simulink library "Nibble_Multiplexers_Lib"  (Simulink 8.7)
settings: Solver=ode45  StartTime=0.0  StopTime=10.0  RelTol=1e-3
libraries: Bit_Multiplexers_Lib x20, commutil2 x16
(part 2 of 2)

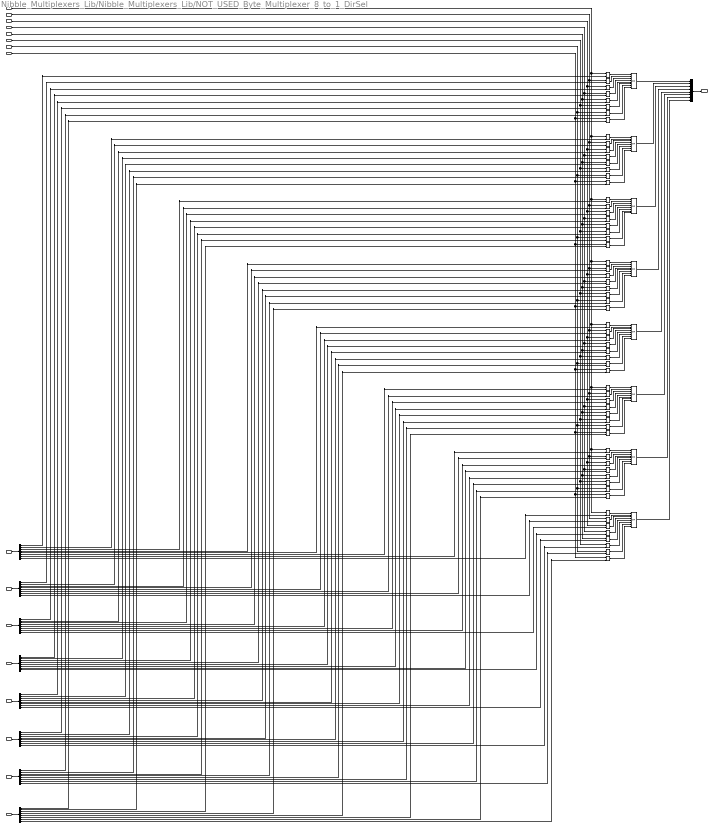
== system Nibble_Multiplexers_Lib/Nibble_Multiplexers_Lib/NOT_USED_Byte_Multiplexer_8_to_1_DirSel ==
  note: Bit_Multiplexer_8_to_1_DirSel(Bit_7)
  note: Bit_Multiplexer_8_to_1_DirSel(Bit_6)
  note: Bit_Multiplexer_8_to_1_DirSel(Bit_5)
  note: Bit_Multiplexer_8_to_1_DirSel(Bit_4)
  note: Bit_Multiplexer_8_to_1_DirSel(Bit_3)
  note: Bit_Multiplexer_8_to_1_DirSel(Bit_2)
  note: Bit_Multiplexer_8_to_1_DirSel(Bit_1)
  note: Bit_Multiplexer_8_to_1_DirSel(Bit_0)
  Select_7(1b) : Inport
  Select_6(1b) : Inport  Port=2
  Select_5(1b) : Inport  Port=3
  Select_4(1b) : Inport  Port=4
  Select_3(1b) : Inport  Port=5
  Select_2(1b) : Inport  Port=6
  Select_1(1b) : Inport  Port=7
  Select_0(1b) : Inport  Port=8
  Data_7(1B) : Inport  Port=9
  Data_6(1B) : Inport  Port=10
  Data_5(1B) : Inport  Port=11
  Data_4(1B) : Inport  Port=12
  Data_3(1B) : Inport  Port=13
  Data_2(1B) : Inport  Port=14
  Data_1(1B) : Inport  Port=15
  Data_0(1B) : Inport  Port=16
  Bus Creator : BusCreator  Inputs=8
  Bus Selector{1..8} (8 alike) : BusSelector  OutputSignals=signal1,signal2,signal3,signal4,signal5,signal6,signal7,signal8
  Logical Operator{,1..7,9..16,18..24,26..33,35..42,44..51,53..60,62..69,71} (64 alike) : Logic  IconShape=distinctive  AllPortsSameDT=off  OutDataTypeStr=boolean
  Logical Operator{8,17,25,34,43,52,61,70} (8 alike) : Logic  Operator=OR  Inputs=8  IconShape=distinctive  OutDataTypeStr=boolean
  Data(1B) : Outport
  wires:
  Data_7(1B)/1 -> Bus Selector7/1
  Bus Creator/1 -> Data(1B)/1
  Bus Selector8/8 -> Logical Operator69/2  "<signal8>"
  Bus Selector6/8 -> Logical Operator68/2  "<signal8>"
  Bus Selector5/8 -> Logical Operator67/2  "<signal8>"
  Bus Selector4/8 -> Logical Operator66/2  "<signal8>"
  Bus Selector3/8 -> Logical Operator65/2  "<signal8>"
  Bus Selector2/8 -> Logical Operator64/2  "<signal8>"
  Bus Selector1/8 -> Logical Operator63/2  "<signal8>"
  Bus Selector7/8 -> Logical Operator71/2  "<signal8>"
  Bus Selector8/7 -> Logical Operator60/2  "<signal7>"
  Bus Selector6/7 -> Logical Operator59/2  "<signal7>"
  Bus Selector5/7 -> Logical Operator58/2  "<signal7>"
  Bus Selector4/7 -> Logical Operator57/2  "<signal7>"
  Bus Selector3/7 -> Logical Operator56/2  "<signal7>"
  Bus Selector2/7 -> Logical Operator55/2  "<signal7>"
  Bus Selector1/7 -> Logical Operator54/2  "<signal7>"
  Bus Selector7/7 -> Logical Operator62/2  "<signal7>"
  Bus Selector8/6 -> Logical Operator51/2  "<signal6>"
  Bus Selector6/6 -> Logical Operator50/2  "<signal6>"
  Bus Selector5/6 -> Logical Operator49/2  "<signal6>"
  Bus Selector4/6 -> Logical Operator48/2  "<signal6>"
  Bus Selector3/6 -> Logical Operator47/2  "<signal6>"
  Bus Selector2/6 -> Logical Operator46/2  "<signal6>"
  Bus Selector1/6 -> Logical Operator45/2  "<signal6>"
  Bus Selector7/6 -> Logical Operator53/2  "<signal6>"
  Bus Selector8/5 -> Logical Operator42/2  "<signal5>"
  Bus Selector6/5 -> Logical Operator41/2  "<signal5>"
  Bus Selector5/5 -> Logical Operator40/2  "<signal5>"
  Bus Selector4/5 -> Logical Operator39/2  "<signal5>"
  Bus Selector3/5 -> Logical Operator38/2  "<signal5>"
  Bus Selector2/5 -> Logical Operator37/2  "<signal5>"
  Bus Selector1/5 -> Logical Operator36/2  "<signal5>"
  Bus Selector7/5 -> Logical Operator44/2  "<signal5>"
  Bus Selector8/4 -> Logical Operator33/2  "<signal4>"
  Bus Selector6/4 -> Logical Operator32/2  "<signal4>"
  Bus Selector5/4 -> Logical Operator31/2  "<signal4>"
  Bus Selector4/4 -> Logical Operator30/2  "<signal4>"
  Bus Selector3/4 -> Logical Operator29/2  "<signal4>"
  Bus Selector2/4 -> Logical Operator28/2  "<signal4>"
  Bus Selector1/4 -> Logical Operator27/2  "<signal4>"
  Bus Selector7/4 -> Logical Operator35/2  "<signal4>"
  Bus Selector8/3 -> Logical Operator24/2  "<signal3>"
  Bus Selector6/3 -> Logical Operator23/2  "<signal3>"
  Bus Selector5/3 -> Logical Operator22/2  "<signal3>"
  Bus Selector4/3 -> Logical Operator21/2  "<signal3>"
  Bus Selector3/3 -> Logical Operator20/2  "<signal3>"
  Bus Selector2/3 -> Logical Operator19/2  "<signal3>"
  Bus Selector1/3 -> Logical Operator18/2  "<signal3>"
  Bus Selector7/3 -> Logical Operator26/2  "<signal3>"
  Bus Selector8/2 -> Logical Operator16/2  "<signal2>"
  Bus Selector6/2 -> Logical Operator15/2  "<signal2>"
  Bus Selector5/2 -> Logical Operator14/2  "<signal2>"
  Bus Selector4/2 -> Logical Operator13/2  "<signal2>"
  Bus Selector3/2 -> Logical Operator12/2  "<signal2>"
  Bus Selector2/2 -> Logical Operator11/2  "<signal2>"
  Bus Selector1/2 -> Logical Operator10/2  "<signal2>"
  Bus Selector7/2 -> Logical Operator9/2  "<signal2>"
  Bus Selector8/1 -> Logical Operator7/2  "<signal1>"
  Bus Selector6/1 -> Logical Operator6/2  "<signal1>"
  Bus Selector5/1 -> Logical Operator5/2  "<signal1>"
  Bus Selector4/1 -> Logical Operator4/2  "<signal1>"
  Bus Selector3/1 -> Logical Operator3/2  "<signal1>"
  Bus Selector2/1 -> Logical Operator2/2  "<signal1>"
  Bus Selector1/1 -> Logical Operator1/2  "<signal1>"
  Bus Selector7/1 -> Logical Operator/2  "<signal1>"
  Select_7(1b)/1 -> Logical Operator44/1, Logical Operator53/1, Logical Operator62/1, Logical Operator71/1, Logical Operator35/1, Logical Operator26/1, Logical Operator9/1, Logical Operator/1
  Select_6(1b)/1 -> Logical Operator36/1, Logical Operator45/1, Logical Operator54/1, Logical Operator63/1, Logical Operator27/1, Logical Operator18/1, Logical Operator10/1, Logical Operator1/1
  Select_4(1b)/1 -> Logical Operator38/1, Logical Operator47/1, Logical Operator56/1, Logical Operator65/1, Logical Operator29/1, Logical Operator20/1, Logical Operator12/1, Logical Operator3/1
  Select_3(1b)/1 -> Logical Operator39/1, Logical Operator48/1, Logical Operator57/1, Logical Operator66/1, Logical Operator30/1, Logical Operator21/1, Logical Operator13/1, Logical Operator4/1
  Select_2(1b)/1 -> Logical Operator40/1, Logical Operator49/1, Logical Operator58/1, Logical Operator67/1, Logical Operator31/1, Logical Operator22/1, Logical Operator14/1, Logical Operator5/1
  Select_0(1b)/1 -> Logical Operator42/1, Logical Operator51/1, Logical Operator60/1, Logical Operator69/1, Logical Operator33/1, Logical Operator24/1, Logical Operator16/1, Logical Operator7/1
  Logical Operator17/1 -> Bus Creator/2
  Logical Operator34/1 -> Bus Creator/4
  Logical Operator52/1 -> Bus Creator/6
  Logical Operator70/1 -> Bus Creator/8
  Select_1(1b)/1 -> Logical Operator41/1, Logical Operator50/1, Logical Operator59/1, Logical Operator68/1, Logical Operator32/1, Logical Operator23/1, Logical Operator15/1, Logical Operator6/1
  Select_5(1b)/1 -> Logical Operator37/1, Logical Operator46/1, Logical Operator55/1, Logical Operator64/1, Logical Operator28/1, Logical Operator19/1, Logical Operator11/1, Logical Operator2/1
  Logical Operator61/1 -> Bus Creator/7
  Logical Operator43/1 -> Bus Creator/5
  Logical Operator25/1 -> Bus Creator/3
  Logical Operator8/1 -> Bus Creator/1
  Logical Operator3/1 -> Logical Operator8/4
  Logical Operator2/1 -> Logical Operator8/3
  Logical Operator1/1 -> Logical Operator8/2
  Logical Operator/1 -> Logical Operator8/1
  Logical Operator7/1 -> Logical Operator8/8
  Logical Operator6/1 -> Logical Operator8/7
  Logical Operator5/1 -> Logical Operator8/6
  Logical Operator4/1 -> Logical Operator8/5
  Logical Operator12/1 -> Logical Operator17/4
  Logical Operator11/1 -> Logical Operator17/3
  Logical Operator10/1 -> Logical Operator17/2
  Logical Operator9/1 -> Logical Operator17/1
  Logical Operator16/1 -> Logical Operator17/8
  Logical Operator15/1 -> Logical Operator17/7
  Logical Operator14/1 -> Logical Operator17/6
  Logical Operator13/1 -> Logical Operator17/5
  Logical Operator20/1 -> Logical Operator25/4
  Logical Operator19/1 -> Logical Operator25/3
  Logical Operator18/1 -> Logical Operator25/2
  Logical Operator26/1 -> Logical Operator25/1
  Logical Operator24/1 -> Logical Operator25/8
  Logical Operator23/1 -> Logical Operator25/7
  Logical Operator22/1 -> Logical Operator25/6
  Logical Operator21/1 -> Logical Operator25/5
  Logical Operator29/1 -> Logical Operator34/4
  Logical Operator28/1 -> Logical Operator34/3
  Logical Operator27/1 -> Logical Operator34/2
  Logical Operator35/1 -> Logical Operator34/1
  Logical Operator33/1 -> Logical Operator34/8
  Logical Operator32/1 -> Logical Operator34/7
  Logical Operator31/1 -> Logical Operator34/6
  Logical Operator30/1 -> Logical Operator34/5
  Logical Operator38/1 -> Logical Operator43/4
  Logical Operator37/1 -> Logical Operator43/3
  Logical Operator36/1 -> Logical Operator43/2
  Logical Operator44/1 -> Logical Operator43/1
  Logical Operator42/1 -> Logical Operator43/8
  Logical Operator41/1 -> Logical Operator43/7
  Logical Operator40/1 -> Logical Operator43/6
  Logical Operator39/1 -> Logical Operator43/5
  Logical Operator47/1 -> Logical Operator52/4
  Logical Operator46/1 -> Logical Operator52/3
  Logical Operator45/1 -> Logical Operator52/2
  Logical Operator53/1 -> Logical Operator52/1
  Logical Operator51/1 -> Logical Operator52/8
  Logical Operator50/1 -> Logical Operator52/7
  Logical Operator49/1 -> Logical Operator52/6
  Logical Operator48/1 -> Logical Operator52/5
  Logical Operator56/1 -> Logical Operator61/4
  Logical Operator55/1 -> Logical Operator61/3
  Logical Operator54/1 -> Logical Operator61/2
  Logical Operator62/1 -> Logical Operator61/1
  Logical Operator60/1 -> Logical Operator61/8
  Logical Operator59/1 -> Logical Operator61/7
  Logical Operator58/1 -> Logical Operator61/6
  Logical Operator57/1 -> Logical Operator61/5
  Logical Operator65/1 -> Logical Operator70/4
  Logical Operator64/1 -> Logical Operator70/3
  Logical Operator63/1 -> Logical Operator70/2
  Logical Operator71/1 -> Logical Operator70/1
  Logical Operator69/1 -> Logical Operator70/8
  Logical Operator68/1 -> Logical Operator70/7
  Logical Operator67/1 -> Logical Operator70/6
  Logical Operator66/1 -> Logical Operator70/5
  Data_0(1B)/1 -> Bus Selector8/1
  Data_1(1B)/1 -> Bus Selector6/1
  Data_2(1B)/1 -> Bus Selector5/1
  Data_3(1B)/1 -> Bus Selector4/1
  Data_4(1B)/1 -> Bus Selector3/1
  Data_5(1B)/1 -> Bus Selector2/1
  Data_6(1B)/1 -> Bus Selector1/1

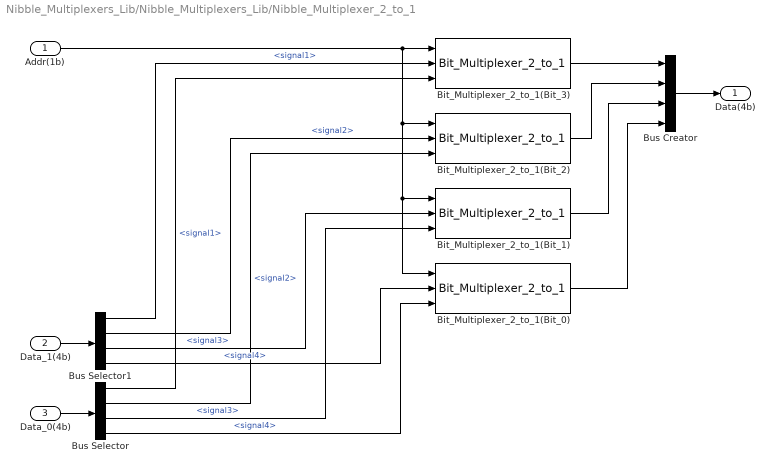
== system Nibble_Multiplexers_Lib/Nibble_Multiplexers_Lib/Nibble_Multiplexer_2_to_1 ==
  Addr(1b) : Inport
  Data_1(4b) : Inport  Port=2
  Data_0(4b) : Inport  Port=3
  Bit_Multiplexer_2_to_1(Bit_0) : Bit_Multiplexers_Lib/Bit_Multiplexers_Lib/Bit_Multiplexer_2_to_1
  Bit_Multiplexer_2_to_1(Bit_1) : Bit_Multiplexers_Lib/Bit_Multiplexers_Lib/Bit_Multiplexer_2_to_1
  Bit_Multiplexer_2_to_1(Bit_2) : Bit_Multiplexers_Lib/Bit_Multiplexers_Lib/Bit_Multiplexer_2_to_1
  Bit_Multiplexer_2_to_1(Bit_3) : Bit_Multiplexers_Lib/Bit_Multiplexers_Lib/Bit_Multiplexer_2_to_1
  Bus Creator : BusCreator  Inputs=4
  Bus Selector : BusSelector  OutputSignals=signal1,signal2,signal3,signal4
  Bus Selector1 : BusSelector  OutputSignals=signal1,signal2,signal3,signal4
  Data(4b) : Outport
  wires:
  Bus Creator/1 -> Data(4b)/1
  Addr(1b)/1 -> Bit_Multiplexer_2_to_1(Bit_3)/1, Bit_Multiplexer_2_to_1(Bit_0)/1, Bit_Multiplexer_2_to_1(Bit_1)/1, Bit_Multiplexer_2_to_1(Bit_2)/1
  Bit_Multiplexer_2_to_1(Bit_0)/1 -> Bus Creator/4
  Bit_Multiplexer_2_to_1(Bit_1)/1 -> Bus Creator/3
  Bit_Multiplexer_2_to_1(Bit_2)/1 -> Bus Creator/2
  Bit_Multiplexer_2_to_1(Bit_3)/1 -> Bus Creator/1
  Data_1(4b)/1 -> Bus Selector1/1
  Data_0(4b)/1 -> Bus Selector/1
  Bus Selector/4 -> Bit_Multiplexer_2_to_1(Bit_0)/3  "<signal4>"
  Bus Selector1/4 -> Bit_Multiplexer_2_to_1(Bit_0)/2  "<signal4>"
  Bus Selector1/3 -> Bit_Multiplexer_2_to_1(Bit_1)/2  "<signal3>"
  Bus Selector/3 -> Bit_Multiplexer_2_to_1(Bit_1)/3  "<signal3>"
  Bus Selector1/2 -> Bit_Multiplexer_2_to_1(Bit_2)/2  "<signal2>"
  Bus Selector/2 -> Bit_Multiplexer_2_to_1(Bit_2)/3  "<signal2>"
  Bus Selector/1 -> Bit_Multiplexer_2_to_1(Bit_3)/3  "<signal1>"
  Bus Selector1/1 -> Bit_Multiplexer_2_to_1(Bit_3)/2  "<signal1>"

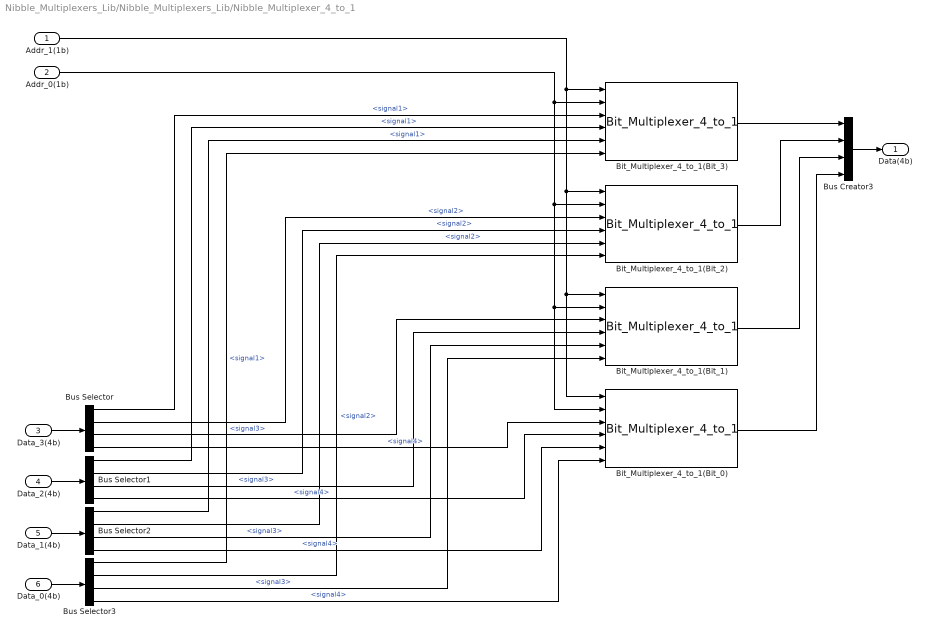
== system Nibble_Multiplexers_Lib/Nibble_Multiplexers_Lib/Nibble_Multiplexer_4_to_1 ==
  Addr_1(1b) : Inport
  Addr_0(1b) : Inport  Port=2
  Data_3(4b) : Inport  Port=3
  Data_2(4b) : Inport  Port=4
  Data_1(4b) : Inport  Port=5
  Data_0(4b) : Inport  Port=6
  Bit_Multiplexer_4_to_1(Bit_0) : Bit_Multiplexers_Lib/Bit_Multiplexers_Lib/Bit_Multiplexer_4_to_1
  Bit_Multiplexer_4_to_1(Bit_1) : Bit_Multiplexers_Lib/Bit_Multiplexers_Lib/Bit_Multiplexer_4_to_1
  Bit_Multiplexer_4_to_1(Bit_2) : Bit_Multiplexers_Lib/Bit_Multiplexers_Lib/Bit_Multiplexer_4_to_1
  Bit_Multiplexer_4_to_1(Bit_3) : Bit_Multiplexers_Lib/Bit_Multiplexers_Lib/Bit_Multiplexer_4_to_1
  Bus Creator3 : BusCreator  Inputs=4
  Bus Selector{,1..3} (4 alike) : BusSelector  OutputSignals=signal1,signal2,signal3,signal4
  Data(4b) : Outport
  wires:
  Bus Creator3/1 -> Data(4b)/1
  Addr_0(1b)/1 -> Bit_Multiplexer_4_to_1(Bit_0)/2, Bit_Multiplexer_4_to_1(Bit_1)/2, Bit_Multiplexer_4_to_1(Bit_2)/2, Bit_Multiplexer_4_to_1(Bit_3)/2
  Addr_1(1b)/1 -> Bit_Multiplexer_4_to_1(Bit_3)/1, Bit_Multiplexer_4_to_1(Bit_0)/1, Bit_Multiplexer_4_to_1(Bit_1)/1, Bit_Multiplexer_4_to_1(Bit_2)/1
  Bit_Multiplexer_4_to_1(Bit_0)/1 -> Bus Creator3/4
  Bit_Multiplexer_4_to_1(Bit_1)/1 -> Bus Creator3/3
  Bit_Multiplexer_4_to_1(Bit_2)/1 -> Bus Creator3/2
  Bit_Multiplexer_4_to_1(Bit_3)/1 -> Bus Creator3/1
  Data_3(4b)/1 -> Bus Selector/1
  Data_2(4b)/1 -> Bus Selector1/1
  Data_1(4b)/1 -> Bus Selector2/1
  Data_0(4b)/1 -> Bus Selector3/1
  Bus Selector/4 -> Bit_Multiplexer_4_to_1(Bit_0)/3  "<signal4>"
  Bus Selector1/4 -> Bit_Multiplexer_4_to_1(Bit_0)/4  "<signal4>"
  Bus Selector2/4 -> Bit_Multiplexer_4_to_1(Bit_0)/5  "<signal4>"
  Bus Selector3/4 -> Bit_Multiplexer_4_to_1(Bit_0)/6  "<signal4>"
  Bus Selector/3 -> Bit_Multiplexer_4_to_1(Bit_1)/3  "<signal3>"
  Bus Selector1/3 -> Bit_Multiplexer_4_to_1(Bit_1)/4  "<signal3>"
  Bus Selector2/3 -> Bit_Multiplexer_4_to_1(Bit_1)/5  "<signal3>"
  Bus Selector3/3 -> Bit_Multiplexer_4_to_1(Bit_1)/6  "<signal3>"
  Bus Selector/2 -> Bit_Multiplexer_4_to_1(Bit_2)/3  "<signal2>"
  Bus Selector1/2 -> Bit_Multiplexer_4_to_1(Bit_2)/4  "<signal2>"
  Bus Selector2/2 -> Bit_Multiplexer_4_to_1(Bit_2)/5  "<signal2>"
  Bus Selector3/2 -> Bit_Multiplexer_4_to_1(Bit_2)/6  "<signal2>"
  Bus Selector/1 -> Bit_Multiplexer_4_to_1(Bit_3)/3  "<signal1>"
  Bus Selector1/1 -> Bit_Multiplexer_4_to_1(Bit_3)/4  "<signal1>"
  Bus Selector2/1 -> Bit_Multiplexer_4_to_1(Bit_3)/5  "<signal1>"
  Bus Selector3/1 -> Bit_Multiplexer_4_to_1(Bit_3)/6  "<signal1>"

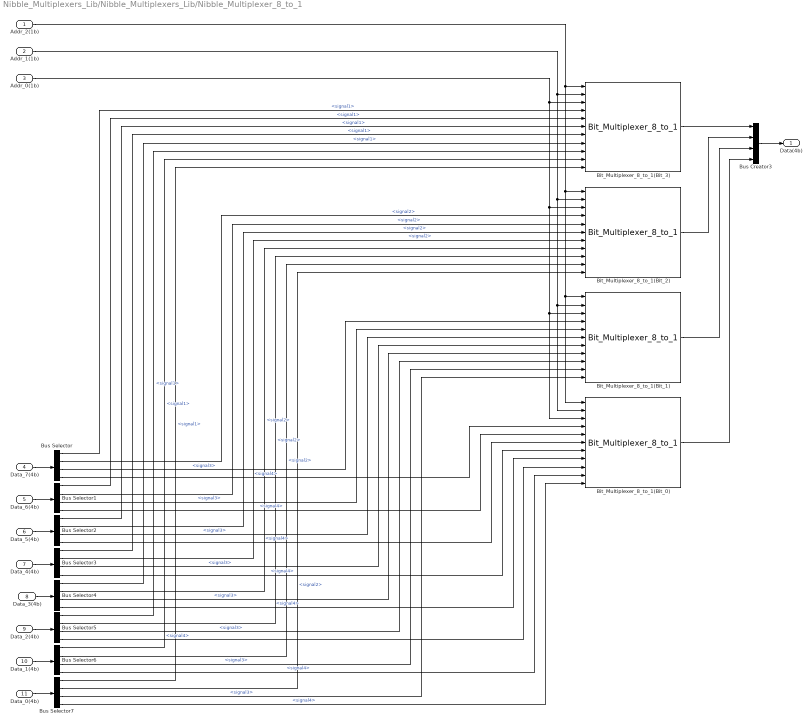
== system Nibble_Multiplexers_Lib/Nibble_Multiplexers_Lib/Nibble_Multiplexer_8_to_1 ==
  Addr_2(1b) : Inport
  Addr_1(1b) : Inport  Port=2
  Addr_0(1b) : Inport  Port=3
  Data_7(4b) : Inport  Port=4
  Data_6(4b) : Inport  Port=5
  Data_5(4b) : Inport  Port=6
  Data_4(4b) : Inport  Port=7
  Data_3(4b) : Inport  Port=8
  Data_2(4b) : Inport  Port=9
  Data_1(4b) : Inport  Port=10
  Data_0(4b) : Inport  Port=11
  Bit_Multiplexer_8_to_1(Bit_0) : Bit_Multiplexers_Lib/Bit_Multiplexers_Lib/Bit_Multiplexer_8_to_1
  Bit_Multiplexer_8_to_1(Bit_1) : Bit_Multiplexers_Lib/Bit_Multiplexers_Lib/Bit_Multiplexer_8_to_1
  Bit_Multiplexer_8_to_1(Bit_2) : Bit_Multiplexers_Lib/Bit_Multiplexers_Lib/Bit_Multiplexer_8_to_1
  Bit_Multiplexer_8_to_1(Bit_3) : Bit_Multiplexers_Lib/Bit_Multiplexers_Lib/Bit_Multiplexer_8_to_1
  Bus Creator3 : BusCreator  Inputs=4
  Bus Selector{,1..7} (8 alike) : BusSelector  OutputSignals=signal1,signal2,signal3,signal4
  Data(4b) : Outport
  wires:
  Bus Creator3/1 -> Data(4b)/1
  Addr_0(1b)/1 -> Bit_Multiplexer_8_to_1(Bit_0)/3, Bit_Multiplexer_8_to_1(Bit_1)/3, Bit_Multiplexer_8_to_1(Bit_2)/3, Bit_Multiplexer_8_to_1(Bit_3)/3
  Addr_1(1b)/1 -> Bit_Multiplexer_8_to_1(Bit_1)/2, Bit_Multiplexer_8_to_1(Bit_0)/2, Bit_Multiplexer_8_to_1(Bit_2)/2, Bit_Multiplexer_8_to_1(Bit_3)/2
  Addr_2(1b)/1 -> Bit_Multiplexer_8_to_1(Bit_0)/1, Bit_Multiplexer_8_to_1(Bit_1)/1, Bit_Multiplexer_8_to_1(Bit_2)/1, Bit_Multiplexer_8_to_1(Bit_3)/1
  Bit_Multiplexer_8_to_1(Bit_0)/1 -> Bus Creator3/4
  Bit_Multiplexer_8_to_1(Bit_1)/1 -> Bus Creator3/3
  Bit_Multiplexer_8_to_1(Bit_2)/1 -> Bus Creator3/2
  Bit_Multiplexer_8_to_1(Bit_3)/1 -> Bus Creator3/1
  Data_7(4b)/1 -> Bus Selector/1
  Data_6(4b)/1 -> Bus Selector1/1
  Data_5(4b)/1 -> Bus Selector2/1
  Data_4(4b)/1 -> Bus Selector3/1
  Data_3(4b)/1 -> Bus Selector4/1
  Data_2(4b)/1 -> Bus Selector5/1
  Data_1(4b)/1 -> Bus Selector6/1
  Data_0(4b)/1 -> Bus Selector7/1
  Bus Selector/1 -> Bit_Multiplexer_8_to_1(Bit_3)/4  "<signal1>"
  Bus Selector1/1 -> Bit_Multiplexer_8_to_1(Bit_3)/5  "<signal1>"
  Bus Selector2/1 -> Bit_Multiplexer_8_to_1(Bit_3)/6  "<signal1>"
  Bus Selector3/1 -> Bit_Multiplexer_8_to_1(Bit_3)/7  "<signal1>"
  Bus Selector4/1 -> Bit_Multiplexer_8_to_1(Bit_3)/8  "<signal1>"
  Bus Selector5/1 -> Bit_Multiplexer_8_to_1(Bit_3)/9  "<signal1>"
  Bus Selector6/1 -> Bit_Multiplexer_8_to_1(Bit_3)/10  "<signal1>"
  Bus Selector7/1 -> Bit_Multiplexer_8_to_1(Bit_3)/11  "<signal1>"
  Bus Selector/2 -> Bit_Multiplexer_8_to_1(Bit_2)/4  "<signal2>"
  Bus Selector1/2 -> Bit_Multiplexer_8_to_1(Bit_2)/5  "<signal2>"
  Bus Selector2/2 -> Bit_Multiplexer_8_to_1(Bit_2)/6  "<signal2>"
  Bus Selector3/2 -> Bit_Multiplexer_8_to_1(Bit_2)/7  "<signal2>"
  Bus Selector4/2 -> Bit_Multiplexer_8_to_1(Bit_2)/8  "<signal2>"
  Bus Selector5/2 -> Bit_Multiplexer_8_to_1(Bit_2)/9  "<signal2>"
  Bus Selector6/2 -> Bit_Multiplexer_8_to_1(Bit_2)/10  "<signal2>"
  Bus Selector7/2 -> Bit_Multiplexer_8_to_1(Bit_2)/11  "<signal2>"
  Bus Selector/3 -> Bit_Multiplexer_8_to_1(Bit_1)/4  "<signal3>"
  Bus Selector1/3 -> Bit_Multiplexer_8_to_1(Bit_1)/5  "<signal3>"
  Bus Selector2/3 -> Bit_Multiplexer_8_to_1(Bit_1)/6  "<signal3>"
  Bus Selector3/3 -> Bit_Multiplexer_8_to_1(Bit_1)/7  "<signal3>"
  Bus Selector4/3 -> Bit_Multiplexer_8_to_1(Bit_1)/8  "<signal3>"
  Bus Selector5/3 -> Bit_Multiplexer_8_to_1(Bit_1)/9  "<signal3>"
  Bus Selector6/3 -> Bit_Multiplexer_8_to_1(Bit_1)/10  "<signal3>"
  Bus Selector7/3 -> Bit_Multiplexer_8_to_1(Bit_1)/11  "<signal3>"
  Bus Selector/4 -> Bit_Multiplexer_8_to_1(Bit_0)/4  "<signal4>"
  Bus Selector1/4 -> Bit_Multiplexer_8_to_1(Bit_0)/5  "<signal4>"
  Bus Selector2/4 -> Bit_Multiplexer_8_to_1(Bit_0)/6  "<signal4>"
  Bus Selector3/4 -> Bit_Multiplexer_8_to_1(Bit_0)/7  "<signal4>"
  Bus Selector4/4 -> Bit_Multiplexer_8_to_1(Bit_0)/8  "<signal4>"
  Bus Selector5/4 -> Bit_Multiplexer_8_to_1(Bit_0)/9  "<signal4>"
  Bus Selector6/4 -> Bit_Multiplexer_8_to_1(Bit_0)/10  "<signal4>"
  Bus Selector7/4 -> Bit_Multiplexer_8_to_1(Bit_0)/11  "<signal4>"
